simulink model "MPC_backend_acados"  (R2026a)
settings: Solver=VariableStepAuto
model workspace (MAT data in the model file):
  kappa_ref = 1
  mpc_ref = 1
undefined symbols (not defined in the file or in its folder): acados_nominal_input
libraries: simulink x1
settings Model: Creator=rayyu  LastModifiedBy=rayyu

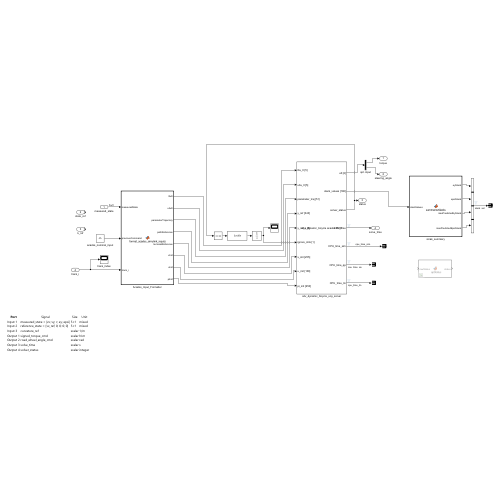
[thumbnail: Simulink's stored preview of the top-level diagram]
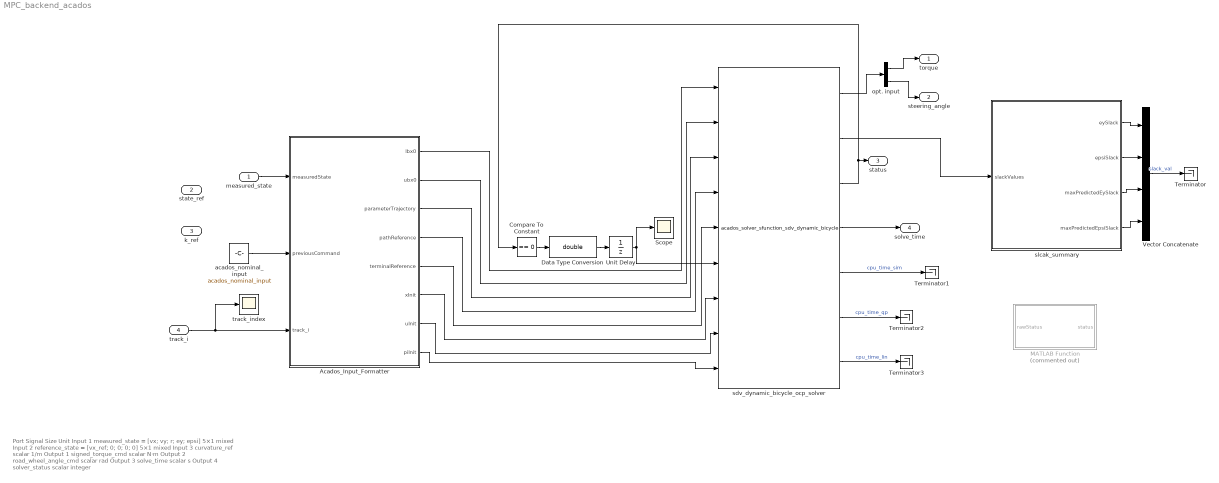
== system MPC_backend_acados ==
  note: Port
      | Signal
      | Size
      | Unit
      |
      | Input 1
      | measured_state = [vx; vy; r; ey; epsi]
      | 5×1
      | mixed
      |
      | Input 2
      | reference_state = [vx_ref; 0; 0; 0; 0]
      | 5×1
      | mixed
      |
      | Input 3
      | curvature_ref
      | scalar
      | 1/m
      |
      | Output 1
      | signed_torque_cmd
      | scalar
      | N·m
      |
      | Output 2
      | road_wheel_angle_cmd
      | scalar
      | rad
      |
      | Output 3
      | solve_time
      | scalar
      | s
      |
      | Output 4
      | solver_status
      | scalar
      | integer
  measured_state : Inport  PortDimensions=[5 1]
  state_ref : Inport  Port=2  PortDimensions=[1 5]
  k_ref : Inport  Port=3  PortDimensions=1
  track_i : Inport  Port=4
  Acados_Input_Formatter : MATLAB Function  TreatAsAtomicUnit=on
  Compare To Constant : simulink/Logic and Bit Operations/Compare To Constant  relop===  const=0  OutDataTypeStr=boolean
  Data Type Conversion : DataTypeConversion  OutDataTypeStr=double  SaturateOnIntegerOverflow=off  RndMeth=Floor
  MATLAB Function : MATLAB Function  Commented=on  TreatAsAtomicUnit=on
  Scope : Scope
      settings: ActiveDisplayYMinimum=-9.5523924081950554E-6  ActiveDisplayYMaximum=1.1223964299354164E-5
  Terminator{,1..3} (4 alike) : Terminator
  Unit Delay : UnitDelay  SampleTime=-1
  Vector Concatenate : Concatenate  NumInputs=4
  acados_nominal_input : Constant  Value=acados_nominal_input  VectorParams1D=off
  opt. input : Demux  Outputs=2
  sdv_dynamic_bicycle_ocp_solver : S-Function  FunctionName=acados_solver_sfunction_sdv_dynamic_bicycle  SFunctionDeploymentMode=off  EnableBusSupport=off
      mask Display:
      | port_label('input', 1, 'lbx_0 [5]')
      | port_label('input', 2, 'ubx_0 [5]')
      | port_label('input', 3, 'parameter_traj [51]')
      | port_label('input', 4, 'y_ref [343]')
      | port_label('input', 5, 'y_ref_e [5]')
      | port_label('input', 6, 'ignore_inits [1]')
      | port_label('input', 7, 'x_init [255]')
      | port_label('input', 8, 'u_init [100]')
      | port_label('input', 9, 'pi_init [250]')
      | port_label('output', 1, 'u0 [2]')
      | port_label('output', 2, 'slack_values [196]')
      | port_label('output', 3, 'solver_status')
      | port_label('output', 4, 'CPU_time')
      | port_label('output', 5, 'CPU_time_sim')
      | port_label('output', 6, 'CPU_time_qp')
      | port_label('output', 7, 'CPU_time_lin')
      | disp('sdv_dynamic_bicycle acados OCP')
  slcak_summary : MATLAB Function  TreatAsAtomicUnit=on
  track_index : Scope
      settings: ActiveDisplayYMinimum=-149.12499999999997  ActiveDisplayYMaximum=1352.125
  torque : Outport
  steering_angle : Outport  Port=2
  status : Outport  Port=3
  solve_time : Outport  Port=4
  wires:
  opt. input/1 -> torque/1
  opt. input/2 -> steering_angle/1
  sdv_dynamic_bicycle_ocp_solver/1 -> opt. input/1
  sdv_dynamic_bicycle_ocp_solver/4 -> solve_time/1
  measured_state/1 -> Acados_Input_Formatter/1(measuredState)
  acados_nominal_input/1 -> Acados_Input_Formatter/2(previousCommand)
  Acados_Input_Formatter/1(lbx0) -> sdv_dynamic_bicycle_ocp_solver/1
  Acados_Input_Formatter/2(ubx0) -> sdv_dynamic_bicycle_ocp_solver/2
  Acados_Input_Formatter/3(parameterTrajectory) -> sdv_dynamic_bicycle_ocp_solver/3
  Acados_Input_Formatter/4(pathReference) -> sdv_dynamic_bicycle_ocp_solver/4
  Acados_Input_Formatter/5(terminalReference) -> sdv_dynamic_bicycle_ocp_solver/5
  sdv_dynamic_bicycle_ocp_solver/3 -> Compare To Constant/1, status/1
  Acados_Input_Formatter/6(xInit) -> sdv_dynamic_bicycle_ocp_solver/7
  Acados_Input_Formatter/7(uInit) -> sdv_dynamic_bicycle_ocp_solver/8
  Acados_Input_Formatter/8(piInit) -> sdv_dynamic_bicycle_ocp_solver/9
  track_i/1 -> track_index/1, Acados_Input_Formatter/3(track_i)
  slcak_summary/1(eySlack) -> Vector Concatenate/1
  slcak_summary/2(epsiSlack) -> Vector Concatenate/2
  slcak_summary/3(maxPredictedEySlack) -> Vector Concatenate/3
  slcak_summary/4(maxPredictedEpsiSlack) -> Vector Concatenate/4
  Vector Concatenate/1 -> Terminator/1  "slack_val"
  Compare To Constant/1 -> Data Type Conversion/1
  Unit Delay/1 -> sdv_dynamic_bicycle_ocp_solver/6, Scope/1
  sdv_dynamic_bicycle_ocp_solver/5 -> Terminator1/1  "cpu_time_sim"
  sdv_dynamic_bicycle_ocp_solver/6 -> Terminator2/1  "cpu_time_qp"
  sdv_dynamic_bicycle_ocp_solver/7 -> Terminator3/1  "cpu_time_lin"
  Data Type Conversion/1 -> Unit Delay/1
  sdv_dynamic_bicycle_ocp_solver/2 -> slcak_summary/1(slackValues)

== matlab function MPC_backend_acados/MATLAB Function ==
  data: rawStatus input; status output
function status = mapStatus(rawStatus)
if rawStatus == 0
    status = 1;
else
    status = -1;
end

end

== matlab function MPC_backend_acados/Acados_Input_Formatter ==
  data: measuredState input; previousCommand input; track_i input; track_ref_table parameter; lbx0 output; ubx0 output; parameterTrajectory output; pathReference output; terminalReference output; xInit output; uInit output; piInit output
function [ ...
    lbx0, ...
    ubx0, ...
    parameterTrajectory, ...
    pathReference, ...
    terminalReference, ...
    xInit, ...
    uInit, ...
    piInit] = ...
    format_acados_simulink_inputs( ...
        measuredState, ...
        previousCommand, ...
        track_i, ...
        track_ref_table)
%FORMAT_ACADOS_SIMULINK_INPUTS Format the N=100 acados S-function inputs.
%
% measuredState   = [vx; vy; yawRate; lateralError; headingError]
% previousCommand = [frontAxleTorque; roadWheelAngle]

numberOfIntervals = 100;
predictionStep_s = 0.01;

%% Fixed-size S-function outputs

lbx0 = zeros(7,1);
ubx0 = zeros(7,1);
parameterTrajectory = zeros(101,1); %#ok<PREALL>
pathReference = zeros(891,1);  % 9*(N-1)
terminalReference = zeros(5,1);
xInit = zeros(707,1);          % 7*(N+1)
uInit = zeros(200,1);          % 2*N
piInit = zeros(700,1);         % 7*N

%% Preview indices for nodes 0 through N

numberOfTrackPoints = size(track_ref_table, 1);
previewIndices = ones(numberOfIntervals + 1, 1);

currentIndex = round(track_i);
currentIndex = max(1, min(currentIndex, numberOfTrackPoints));

previewIndices(1) = currentIndex;
predictedStation_m = track_ref_table(currentIndex, 1);

for node = 2:(numberOfIntervals + 1)

    currentIndex = previewIndices(node - 1);
    predictedSpeed_mps = ...
        max(track_ref_table(currentIndex, 6), 0);

    predictedStation_m = ...
        predictedStation_m ...
        + predictedSpeed_mps*predictionStep_s;

    nextIndex = currentIndex;

    while nextIndex < numberOfTrackPoints && ...
            track_ref_table(nextIndex, 1) < predictedStation_m

        nextIndex = nextIndex + 1;
    end

    previewIndices(node) = nextIndex;
end

%% Curvature preview for nodes 0 through N

for node = 1:(numberOfIntervals + 1)
    parameterTrajectory(node) = ...
        track_ref_table(previewIndices(node), 5);
end

%% Nine-element references for stages 1 through N-1

for stage = 1:(numberOfIntervals - 1)

    referenceIndex = previewIndices(stage + 1);

    stageReference = [
        track_ref_table(referenceIndex, 6)  % vx reference
        0                                   % vy reference
        track_ref_table(referenceIndex, 7)  % yaw-rate reference
        0                                   % lateral-error reference
        0                                   % heading-error reference
        0                                   % torque-effort reference
        0                                   % steering-effort reference
        0                                   % torque-rate reference
        0                                   % steering-rate reference
        ];

    outputStartIndex = (stage - 1)*9 + 1;

    for element = 1:9
        pathReference(outputStartIndex + element - 1) = ...
            stageReference(element);
    end
end

%% Initial augmented state

for stateIndex = 1:5
    lbx0(stateIndex) = measuredState(stateIndex);
    ubx0(stateIndex) = measuredState(stateIndex);
end

for commandIndex = 1:2
    lbx0(5 + commandIndex) = previousCommand(commandIndex);
    ubx0(5 + commandIndex) = previousCommand(commandIndex);
end

%% Terminal reference contains only the five vehicle states

terminalIndex = previewIndices(numberOfIntervals + 1);

terminalReference = [
    track_ref_table(terminalIndex, 6)
    0
    track_ref_table(terminalIndex, 7)
    0
    0
    ];

%% External state-trajectory initialization

for stage = 0:numberOfIntervals

    startIndex = stage*7 + 1;

    for stateIndex = 1:5
        xInit(startIndex + stateIndex - 1) = ...
            measuredState(stateIndex);
    end

    xInit(startIndex + 5) = previousCommand(1);
    xInit(startIndex + 6) = previousCommand(2);
end

% uInit and piInit intentionally remain zero. The optimizer inputs are
% command rates, so zero is the neutral cold-start guess.

end

== matlab function MPC_backend_acados/slcak_summary ==
  data: slackValues input; eySlack output; epsiSlack output; maxPredictedEySlack output; maxPredictedEpsiSlack output
function [eySlack, epsiSlack, ...
          maxPredictedEySlack, ...
          maxPredictedEpsiSlack] = ...
          summarizeSlacks(slackValues)

% Two states, each having lower and upper slack.
slackByStage = reshape(slackValues, 4, []);

lowerEy   = slackByStage(1,:);
lowerEpsi = slackByStage(2,:);
upperEy   = slackByStage(3,:);
upperEpsi = slackByStage(4,:);

% Violation predicted at the first constrained prediction stage.
eySlack = max(lowerEy(1), upperEy(1));
epsiSlack = max(lowerEpsi(1), upperEpsi(1));

% Largest violation anywhere in the current prediction horizon.
maxPredictedEySlack = ...
    max(max(lowerEy, upperEy));

maxPredictedEpsiSlack = ...
    max(max(lowerEpsi, upperEpsi));

end
